simulink model "model4_3_2"  (R2019b)
settings: Solver=VariableStepAuto  StartTime=0.0  StopTime=10.0  RelTol=1e-3
values from neighbouring files (symbols this model uses):
  a1 = 2    [lab4_3.m]
  a2 = 3    [lab4_3.m]
  a3 = 1    [lab4_3.m]
  a4 = 2    [lab4_3.m]
  a5 = 4    [lab4_3.m]
  f1 = 1    [lab4_3.m]
  f2 = 5    [lab4_3.m]
  f3 = 2    [lab4_3.m]
  f4 = 1    [lab4_3.m]
  f5 = 0    [lab4_3.m]
  w1 = 0.001    [lab4_3.m]
  w2 = 1    [lab4_3.m]
  w3 = 30    [lab4_3.m]
  w4 = 0.01    [lab4_3.m]
  w5 = 5    [lab4_3.m]
settings Model: Creator=marci  LastModifiedBy=marci

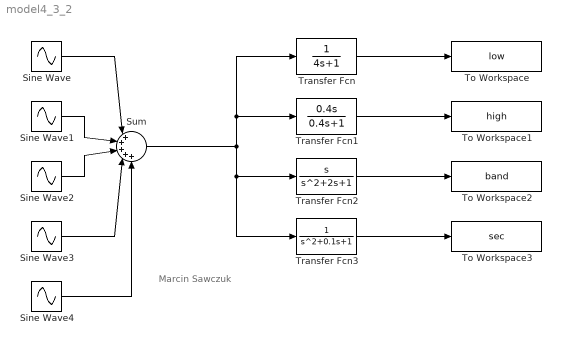
== system model4_3_2 ==
  note: Marcin Sawczuk
  Sine Wave : Sin  Amplitude=a1  Frequency=w1  Phase=f1  SampleTime=0
  Sine Wave1 : Sin  Amplitude=a2  Frequency=w2  Phase=f2  SampleTime=0
  Sine Wave2 : Sin  Amplitude=a3  Frequency=w3  Phase=f3  SampleTime=0
  Sine Wave3 : Sin  Amplitude=a4  Frequency=w4  Phase=f4  SampleTime=0
  Sine Wave4 : Sin  Amplitude=a5  Frequency=w5  Phase=f5  SampleTime=0
  Sum : Sum  Inputs=|+++++
  To Workspace : ToWorkspace  VariableName=low  SaveFormat=Timeseries  SampleTime=-1
  To Workspace1 : ToWorkspace  VariableName=high  SaveFormat=Timeseries  SampleTime=-1
  To Workspace2 : ToWorkspace  VariableName=band  SaveFormat=Timeseries  SampleTime=-1
  To Workspace3 : ToWorkspace  VariableName=sec  SaveFormat=Timeseries  SampleTime=-1
  Transfer Fcn : TransferFcn  Denominator=[4 1]
  Transfer Fcn1 : TransferFcn  Numerator=[0.4 0]  Denominator=[0.4 1]
  Transfer Fcn2 : TransferFcn  Numerator=[1 0]
  Transfer Fcn3 : TransferFcn  Denominator=[1 0.1 1]
  wires:
  Transfer Fcn/1 -> To Workspace/1
  Transfer Fcn1/1 -> To Workspace1/1
  Transfer Fcn2/1 -> To Workspace2/1
  Transfer Fcn3/1 -> To Workspace3/1
  Sum/1 -> Transfer Fcn3/1, Transfer Fcn2/1, Transfer Fcn1/1, Transfer Fcn/1
  Sine Wave/1 -> Sum/1
  Sine Wave1/1 -> Sum/2
  Sine Wave2/1 -> Sum/3
  Sine Wave3/1 -> Sum/4
  Sine Wave4/1 -> Sum/5
